simulink model "ACS"  (R2024b)
settings: Solver=FixedStepDiscrete  StartTime=0.0  StopTime=10.0  FixedStep=.01  RelTol=1e-3
libraries: simulink x1
settings DataIOCC: LoggingToFile=on
settings DebuggingCC: AlgebraicLoopMsg=error

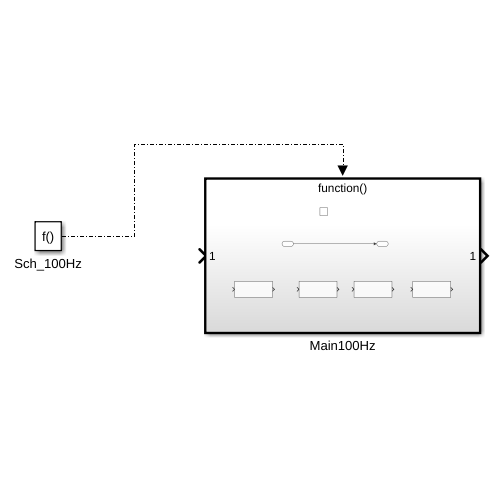
[thumbnail: Simulink's stored preview of the top-level diagram]
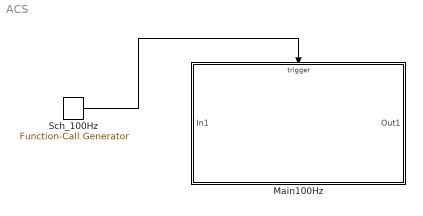
== system ACS ==
  Main100Hz : Subsystem  TreatAsAtomicUnit=on
  Sch_100Hz : simulink/Ports & Subsystems/Function-Call Generator  sample_time=0.01  numberOfIterations=1  DisallowWideOutput=off
  wires:
  Sch_100Hz/1 -> Main100Hz/Trigger

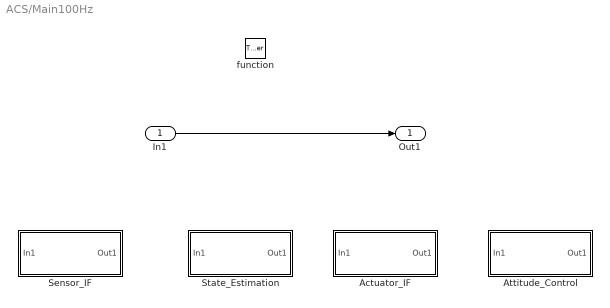
== system ACS/Main100Hz ==
  In1 : Inport
  function : TriggerPort  TriggerType=function-call  VariantControl=(inherit)
  Actuator_IF : Subsystem
  Attitude_Control : Subsystem
  Sensor_IF : Subsystem
  State_Estimation : Subsystem
  Out1 : Outport
  wires:
  In1/1 -> Out1/1

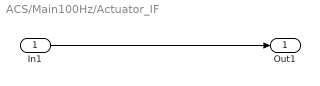
== system ACS/Main100Hz/Actuator_IF ==
  In1 : Inport
  Out1 : Outport
  wires:
  In1/1 -> Out1/1

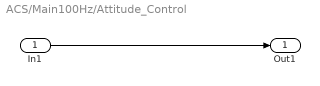
== system ACS/Main100Hz/Attitude_Control ==
  In1 : Inport
  Out1 : Outport
  wires:
  In1/1 -> Out1/1

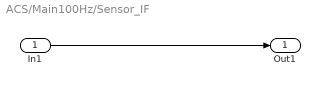
== system ACS/Main100Hz/Sensor_IF ==
  In1 : Inport
  Out1 : Outport  OutDataTypeStr=Bus: IMUBus
  wires:
  In1/1 -> Out1/1

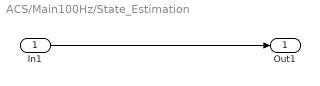
== system ACS/Main100Hz/State_Estimation ==
  In1 : Inport
  Out1 : Outport
  wires:
  In1/1 -> Out1/1
